simulink model "G_complete"  (R2020b)
settings: Solver=VariableStepAuto  StartTime=0.0  StopTime=2  RelTol=1e-9
undefined symbols (not defined in the file or in its folder): K_adc, K_lvdt, T_i
libraries: cstblocks x8
settings Model: Creator=jasper  LastModifiedBy=jasper

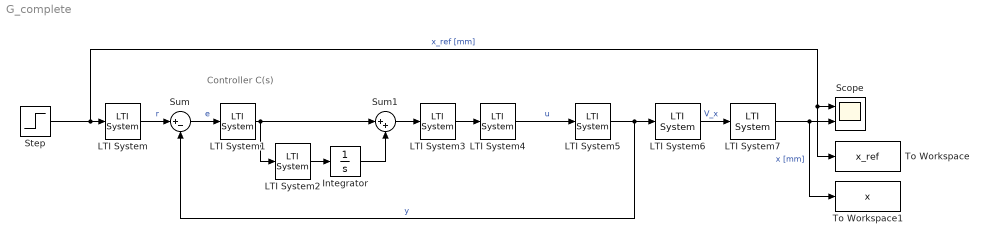
== system G_complete ==
  note: Controller C(s)
  Integrator : Integrator  LimitOutput=on  UpperSaturationLimit=10  LowerSaturationLimit=-10
  LTI System : cstblocks/LTI System  sys=H  IC=[]
  LTI System1 : cstblocks/LTI System  sys=K_p  IC=[]
  LTI System2 : cstblocks/LTI System  sys=1/T_i  IC=[]
  LTI System3 : cstblocks/LTI System  sys=G_lead  IC=[]
  LTI System4 : cstblocks/LTI System  sys=G_lpf  IC=[]
  LTI System5 : cstblocks/LTI System  sys=P  IC=[]
  LTI System6 : cstblocks/LTI System  sys=1/K_adc  IC=[]
  LTI System7 : cstblocks/LTI System  sys=1/K_lvdt  IC=[]
  Scope : Scope  NumInputPorts=2
  Step : Step  Time=0.1  SampleTime=0
  Sum : Sum  Inputs=|+-
  Sum1 : Sum  Inputs=|++
  To Workspace : ToWorkspace  VariableName=x_ref  SaveFormat=Timeseries  SampleTime=-1
  To Workspace1 : ToWorkspace  VariableName=x  SaveFormat=Timeseries  SampleTime=-1
  wires:
  Step/1 -> Scope/1, To Workspace/1, LTI System/1  "x_ref [mm]"
  LTI System/1 -> Sum/1  "r"
  Sum/1 -> LTI System1/1  "e"
  LTI System1/1 -> Sum1/1, LTI System2/1
  LTI System2/1 -> Integrator/1
  Integrator/1 -> Sum1/2
  Sum1/1 -> LTI System3/1
  LTI System3/1 -> LTI System4/1
  LTI System4/1 -> LTI System5/1  "u"
  LTI System5/1 -> Sum/2, LTI System6/1  "y"
  LTI System7/1 -> To Workspace1/1, Scope/2  "x [mm]"
  LTI System6/1 -> LTI System7/1  "V_x"
